simulink model "sistema"  (R2025a)
settings: Solver=VariableStepAuto  StartTime=0.0  StopTime=10.0  MaxStep=1e-3  RelTol=1e-3
libraries: slpidlib x1, simulink x1
settings DataIOCC: ReturnWorkspaceOutputs=off  TimeSaveName=t
settings DebuggingCC: AlgebraicLoopMsg=none  ArtificialAlgebraicLoopMsg=none  MaxConsecutiveZCsMsg=none

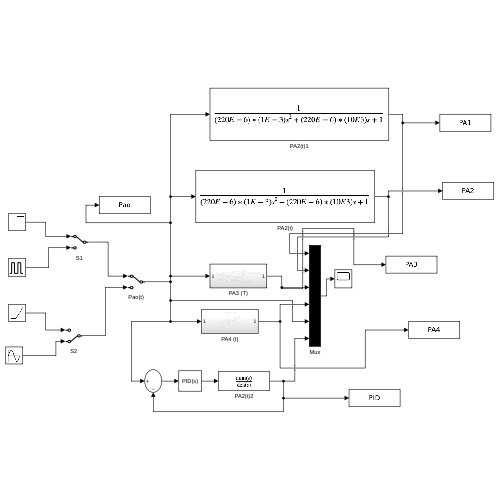
[thumbnail: Simulink's stored preview of the top-level diagram]
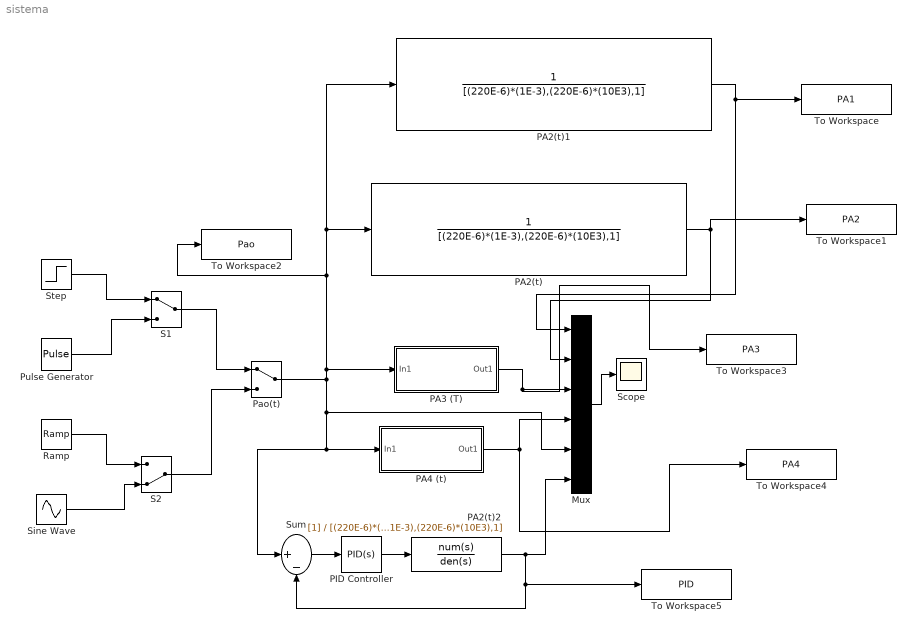
== system sistema ==
  Mux : Mux  Inputs=6
  PA2(t) : TransferFcn  Denominator=[(220E-6)*(1E-3),(220E-6)*(10E3),1]
  PA2(t)1 : TransferFcn  Denominator=[(220E-6)*(1E-3),(220E-6)*(10E3),1]
  PA2(t)2 : TransferFcn  Denominator=[(220E-6)*(1E-3),(220E-6)*(10E3),1]
  PA3 (T) : Subsystem
  PA4 (t) : Subsystem
  PID Controller : slpidlib/PID Controller  Controller=PID  Form=Parallel  TimeDomain=Continuous-time  UseExternalTs=off  SampleTime=-1  IntegratorMethod=Forward Euler  FilterMethod=Forward Euler  ControllerParametersSource=internal  P=289.680927538353  I=7062.47058056347  UseKiTs=off  D=0.391371372630429  UseExternalDerivativeSource=off  N=503.010216106345  UseFilter=on  TunerSelectOption=Transfer Function Based (PID Tuner App)  InitialConditionSource=internal  InitialConditionForIntegrator=0  InitialConditionForFilter=0  DifferentiatorICPrevScaledInput=0  ExternalReset=none  TrackingMode=off  Kt=1  LimitOutput=off  SatLimitsSource=internal  UpperSaturationLimit=inf  LowerSaturationLimit=-inf  LinearizeAsGain=on  AntiWindupMode=none  Kb=1  LimitIntegrator=off  UpperIntegratorSaturationLimit=inf  LowerIntegratorSaturationLimit=-inf  POutMin=[]  POutMax=[]  IOutMin=[]  IOutMax=[]  DOutMin=[]  DOutMax=[]  NOutMin=[]  NOutMax=[]  SumOutMin=[]  SumOutMax=[]  SaturationOutMin=[]  SaturationOutMax=[]  PParamMin=[]  PParamMax=[]  IParamMin=[]  IParamMax=[]  DParamMin=[]  DParamMax=[]  NParamMin=[]  NParamMax=[]  KbParamMin=[]  KbParamMax=[]  KtParamMin=[]  KtParamMax=[]  KbOutMin=[]  KbOutMax=[]  KtOutMin=[]  KtOutMax=[]  IntegratorOutMin=[]  IntegratorOutMax=[]  FilterOutMin=[]  FilterOutMax=[]  SumI1OutMin=[]  SumI1OutMax=[]  SumI2OutMin=[]  SumI2OutMax=[]  SumI3OutMin=[]  SumI3OutMax=[]  SumI4OutMin=[]  SumI4OutMax=[]  SumDOutMin=[]  SumDOutMax=[]  DifferentiatorOutMin=[]  DifferentiatorOutMax=[]  FilterDiffOutCoefMin=[]  FilterDiffOutCoefMax=[]  ReciprocalOutMin=[]  ReciprocalOutMax=[]  SumDenOutMin=[]  SumDenOutMax=[]  SumNumOutMin=[]  SumNumOutMax=[]  DivideOutMin=[]  DivideOutMax=[]  UdiffTsProdOutMin=[]  UdiffTsProdOutMax=[]  NTsProdOutMin=[]  NTsProdOutMax=[]  UintegralTsProdOutMin=[]  UintegralTsProdOutMax=[]  UngainTsProdOutMin=[]  UngainTsProdOutMax=[]  ClampingZeroOutDataTypeStr=Inherit: Inherit via back propagation  ClampingZeroOutMin=[]  ClampingZeroOutMax=[]  FilterDenConstantOutDataTypeStr=Inherit: Inherit via back propagation  FilterDenConstantOutMin=[]  FilterDenConstantOutMax=[]  PCopyOutDataTypeStr=Inherit: Inherit via back propagation  PCopyOutMin=[]  PCopyOutMax=[]  NCopyOutDataTypeStr=Inherit: Inherit via back propagation  NCopyOutMin=[]  NCopyOutMax=[]  IntegratorContinuousStateAttributes=''  IntegratorStateMustResolveToSignalObject=off  IntegratorRTWStateStorageClass=Auto  FilterContinuousStateAttributes=''  FilterStateMustResolveToSignalObject=off  FilterRTWStateStorageClass=Auto  ParallelPVariant=InternalParameters  IdealPVariant=Disabled  IVariant=InternalParameters  DVariant=InternalParameters  IntegratorVariant=Continuous  SatVariant=Disabled  AWVariant=Passthrough  PCopyVariant=Disabled  TRVariant=Disabled  FdbkBlocksVariant=Forward  IdealPFdbkVariant=Disabled  SatFdbkVariant=Disabled  DerivativeFilterVariant=ContFilter  NVariant=InternalParameters  NCopyVariant=Disabled  FilterICVariant=InternalICsFilter  IntegratorICVariant=InternalICs  ExternalResetVariant=Disabled  TRSumVariant=Passthrough  SumFdbkVariant=Disabled  SumVariant=Sum_PID  TsampFilterVariant=InternalTs  TsampNgainVariant=Passthrough  TsampIntegralVariant=Disabled_SignalSpec  ExternalSaturationOutDataTypeStr=Inherit: Same as second input  DerivativeSourceVariant=ErrorSignal  PreIntVariant=InternalPreInt
  Pao(t) : ManualSwitch
  Pulse Generator : DiscretePulseGenerator  PulseType=Time based  Period=10  PulseWidth=10  PhaseDelay=1
  Ramp : simulink/Sources/Ramp  slope=1/10  start=0  InitialOutput=0
  S1 : ManualSwitch
  S2 : ManualSwitch  CurrentSetting=0
  Scope : Scope
      settings: ActiveDisplayYMinimum=-0.12501213344590831  ActiveDisplayYMaximum=1.1251092010131751
  Sine Wave : Sin  Frequency=pi/2  SampleTime=0
  Step : Step  Time=0  Before=1  SampleTime=0
  Sum : Sum  Inputs=|+-
  To Workspace : ToWorkspace  VariableName=PA1  SampleTime=-1
  To Workspace1 : ToWorkspace  VariableName=PA2  SampleTime=-1
  To Workspace2 : ToWorkspace  VariableName=Pao  SampleTime=-1
  To Workspace3 : ToWorkspace  VariableName=PA3  SampleTime=-1
  To Workspace4 : ToWorkspace  VariableName=PA4  SampleTime=-1
  To Workspace5 : ToWorkspace  VariableName=PID  SampleTime=-1
  wires:
  Step/1 -> S1/1
  Pulse Generator/1 -> S1/2
  Ramp/1 -> S2/1
  Sine Wave/1 -> S2/2
  S1/1 -> Pao(t)/1
  S2/1 -> Pao(t)/2
  Pao(t)/1 -> PA3 (T)/1(In1), To Workspace2/1, PA2(t)1/1, PA2(t)/1, Sum/1, PA4 (t)/1(In1), Mux/5
  PA2(t)/1 -> To Workspace1/1, Mux/2
  PA3 (T)/1(Out1) -> To Workspace3/1, Mux/3
  PA4 (t)/1(Out1) -> To Workspace4/1, Mux/4
  Mux/1 -> Scope/1
  PA2(t)1/1 -> To Workspace/1, Mux/1
  Sum/1 -> PID Controller/1
  PID Controller/1 -> PA2(t)2/1
  PA2(t)2/1 -> Mux/6, To Workspace5/1, Sum/2

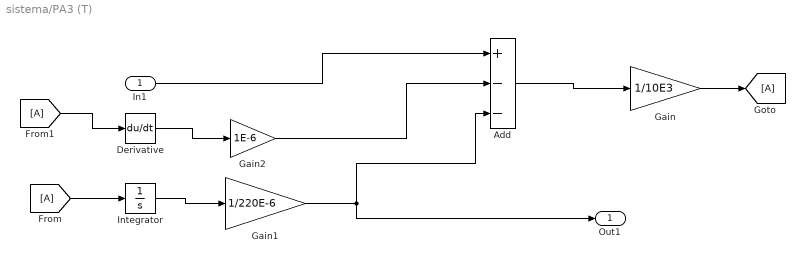
== system sistema/PA3 (T) ==
  In1 : Inport
  Add : Sum  Inputs=+--
  Derivative : Derivative
  From : From
  From1 : From
  Gain : Gain  Gain=1/10E3
  Gain1 : Gain  Gain=1/220E-6
  Gain2 : Gain  Gain=1E-6
  Goto : Goto
  Integrator : Integrator
  Out1 : Outport
  wires:
  In1/1 -> Add/1
  Derivative/1 -> Gain2/1
  Gain2/1 -> Add/2
  Integrator/1 -> Gain1/1
  Gain1/1 -> Out1/1, Add/3
  Add/1 -> Gain/1
  Gain/1 -> Goto/1
  From1/1 -> Derivative/1
  From/1 -> Integrator/1

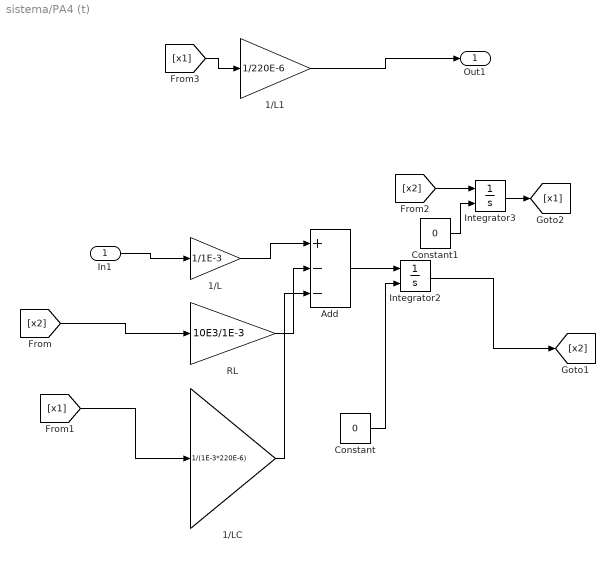
== system sistema/PA4 (t) ==
  In1 : Inport
  1/L : Gain  Gain=1/1E-3
  1/L1 : Gain  Gain=1/220E-6
  1/LC : Gain  Gain=1/(1E-3*220E-6)
  Add : Sum  Inputs=+--
  Constant : Constant  Value=0
  Constant1 : Constant  Value=0
  Integrator2 : Integrator  InitialConditionSource=external
  Integrator3 : Integrator  InitialConditionSource=external
  RL : Gain  Gain=10E3/1E-3
  Out1 : Outport
  wires:
  In1/1 -> 1/L/1
  1/L/1 -> Add/1
  RL/1 -> Add/2
  [x2] -> RL/1
  1/LC/1 -> Add/3
  [x1] -> 1/LC/1
  Add/1 -> Integrator2/1
  Constant/1 -> Integrator2/2
  [x2] -> Integrator3/1
  Constant1/1 -> Integrator3/2
  Integrator3/1 -> [x1]
  Integrator2/1 -> [x2]
  [x1] -> 1/L1/1
  1/L1/1 -> Out1/1
